simulink model "motorcontrol"  (R2020b)
settings: Solver=FixedStepDiscrete  StartTime=0.0  StopTime=20  FixedStep=Ts.simulink  MaxStep=5e-5  RelTol=1e-3  EnableMultiTasking=on
values from neighbouring files (symbols this model uses):
  dataType = 'single'    [motorcontrol_params.m]
undefined symbols (not defined in the file or in its folder): ControllerMode, ControlMode, ctrlParams, DiscIntNeverNeededParam, inverter, NumBits1, NumBits2, PI_params, pmsm, Slope1, Slope2, Ts
libraries: simulink x14, pid_lib x3
(part 1 of 3)
settings Model: Creator=26046633  LastModifiedBy=26046633
settings SolverCC: ZeroCrossAlgorithm=Adaptive
settings OptimizationCC: DefaultUnderspecifiedDataType=single
settings DebuggingCC: IgnoredZcDiagnostic=none  MultiTaskDSMMsg=none  IntegerOverflowMsg=none  ParameterOverflowMsg=none  ParameterPrecisionLossMsg=none  ParameterTunabilityLossMsg=none
settings RTWCC: Toolchain=MinGW64 | gmake (64-bit Windows)

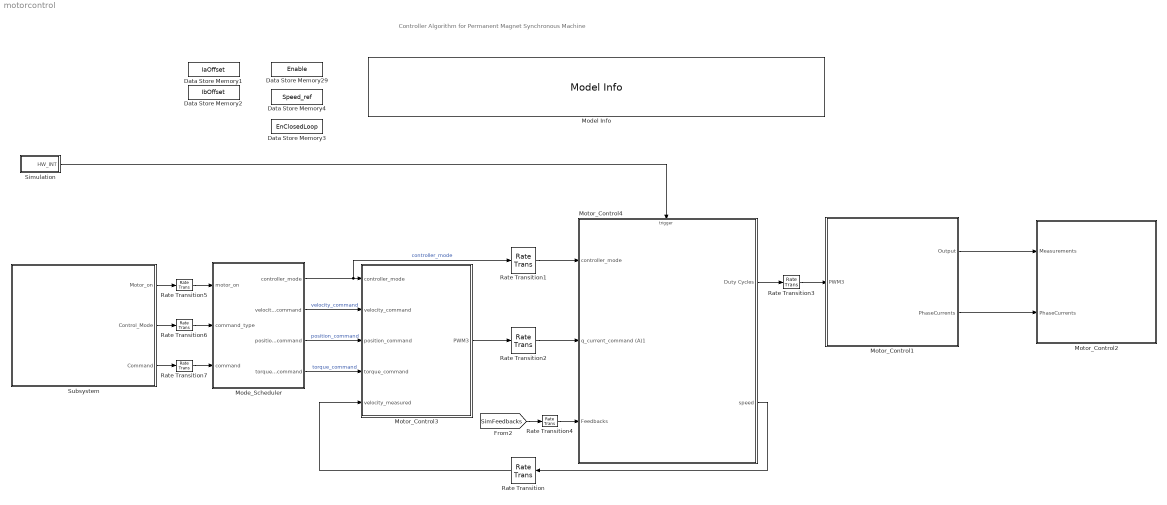
== system motorcontrol ==
  note: Controller Algorithm for Permanent Magnet Synchronous Machine
  Data Store Memory1 : DataStoreMemory  DataStoreName=IaOffset  InitialValue=inverter.CtSensAOffset  ShowAdditionalParam=off
  Data Store Memory2 : DataStoreMemory  DataStoreName=IbOffset  InitialValue=inverter.CtSensBOffset  ShowAdditionalParam=off
  Data Store Memory29 : DataStoreMemory  DataStoreName=Enable  ShowAdditionalParam=off  OutDataTypeStr=boolean
  Data Store Memory3 : DataStoreMemory  DataStoreName=EnClosedLoop  ShowAdditionalParam=off  OutDataTypeStr=boolean
  Data Store Memory4 : DataStoreMemory  DataStoreName=Speed_ref  ShowAdditionalParam=off  OutDataTypeStr=dataType
  Mode_Scheduler : Subsystem  TreatAsAtomicUnit=on  SystemSampleTime=Ts.speed
      mask Display: fprintf('Mode\nScheduler')
  Model Info : simulink/Model-Wide Utilities/Model Info  Frame=on  DisplayStringWithTags=|  HorizontalTextAlignment=Left  LeftAlignmentValue=0.02
      | %<Description>  Model Description: Controller Algorithm for Permanent Magnet Synchronous Motor
      | 
      | %<ModifiedComment> Specifies controller software for Permanent Magnet Synchronous Machine (PMSM) using Field-Oriented Control.
      | 
      | Created By: %<Created>  | Alper Senem [26046633]
      | Last Modification: %<LastModificationDate> | %<LastModifiedBy>
      | Version: %<ModelVersion>
  Motor_Control1 : Subsystem
      settings: RTWSystemCode=Nonreusable function  RTWFcnNameOpts=Use subsystem name
      mask Display: fprintf('Voltage Source Inverter \n\n & PMSM')
  Motor_Control2 : Subsystem
      settings: RTWSystemCode=Nonreusable function  RTWFcnNameOpts=Use subsystem name
      mask Display: fprintf('Measurements')
  Motor_Control3 : Subsystem  TreatAsAtomicUnit=on  SystemSampleTime=Ts.speed
      settings: RTWSystemCode=Nonreusable function  RTWFcnNameOpts=Use subsystem name
      mask Display: fprintf('Motor\nControl')
  Motor_Control4 : Subsystem
      settings: RTWSystemCode=Nonreusable function  RTWFcnNameOpts=Use subsystem name
      mask Display: fprintf('Field Oriented\nControl')
  Rate Transition : RateTransition  Deterministic=off  OutPortSampleTime=Ts.speed
  Rate Transition1 : RateTransition  Deterministic=off  InitialCondition=ControllerMode.SpeedControl  OutPortSampleTime=Ts.pwm
  Rate Transition2 : RateTransition  Deterministic=off  OutPortSampleTime=Ts.pwm
  Rate Transition3 : RateTransition  Deterministic=off  OutPortSampleTime=Ts.inverter
  Rate Transition4 : RateTransition  Deterministic=off  OutPortSampleTime=Ts.pwm
  Rate Transition5 : RateTransition  Integrity=off  Deterministic=off  OutPortSampleTime=Ts.speed
  Rate Transition6 : RateTransition  Integrity=off  Deterministic=off  OutPortSampleTime=Ts.speed
  Rate Transition7 : RateTransition  Deterministic=off  OutPortSampleTime=Ts.speed
  Simulation : Subsystem
  Subsystem : Subsystem  TreatAsAtomicUnit=on  SystemSampleTime=0.01
  wires:
  Motor_Control3/1(PWM3) -> Rate Transition2/1
  Motor_Control1/1(Output) -> Motor_Control2/1(Measurements)
  Motor_Control4/2(speed) -> Rate Transition/1
  Subsystem/3(Command) -> Rate Transition7/1
  Rate Transition/1 -> Motor_Control3/5(velocity_measured)
  Subsystem/2(Control_Mode) -> Rate Transition6/1
  Subsystem/1(Motor_on) -> Rate Transition5/1
  Mode_Scheduler/1(controller_mode) -> Rate Transition1/1, Motor_Control3/1(controller_mode)  "controller_mode"
  Mode_Scheduler/2(velocity_command) -> Motor_Control3/2(velocity_command)  "velocity_command"
  Mode_Scheduler/4(torque_command) -> Motor_Control3/4(torque_command)  "torque_command"
  Mode_Scheduler/3(position_command) -> Motor_Control3/3(position_command)  "position_command"
  Simulation/1(HW_INT) -> Motor_Control4/Trigger
  Motor_Control4/1(Duty Cycles) -> Rate Transition3/1
  Motor_Control1/2(PhaseCurrents) -> Motor_Control2/2(PhaseCurrents)
  Rate Transition3/1 -> Motor_Control1/1(PWM3)
  Rate Transition4/1 -> Motor_Control4/3(Feedbacks)
  Rate Transition2/1 -> Motor_Control4/2(q_current_command (A)1)
  [SimFeedbacks] -> Rate Transition4/1
  Rate Transition1/1 -> Motor_Control4/1(controller_mode)
  Rate Transition5/1 -> Mode_Scheduler/1(motor_on)
  Rate Transition6/1 -> Mode_Scheduler/2(command_type)
  Rate Transition7/1 -> Mode_Scheduler/3(command)

== system motorcontrol/Mode_Scheduler ==
  note: Mode Scheduler
  note: Configures controller mode and controller inputs based on user commands.
  motor_on : Inport
  command_type : Inport  Port=2
  command : Inport  Port=3
  Controller_Mode_Scheduler : Stateflow chart  SystemSampleTime=Ts
  Signal Conversion : SignalConversion  OverrideOpt=on
  Signal Conversion1 : SignalConversion  OverrideOpt=on
  Signal Conversion2 : SignalConversion  OverrideOpt=on
  controller_mode : Outport
  velocity_command : Outport  Port=2
  position_command : Outport  Port=3
  torque_command : Outport  Port=4
  wires:
  Signal Conversion2/1 -> Controller_Mode_Scheduler/3(command)
  Signal Conversion1/1 -> Controller_Mode_Scheduler/2(command_type)
  Signal Conversion/1 -> Controller_Mode_Scheduler/1(motor_on)
  command/1 -> Signal Conversion2/1
  Controller_Mode_Scheduler/4(torque_command) -> torque_command/1
  command_type/1 -> Signal Conversion1/1
  Controller_Mode_Scheduler/3(position_command) -> position_command/1
  motor_on/1 -> Signal Conversion/1
  Controller_Mode_Scheduler/2(velocity_command) -> velocity_command/1
  Controller_Mode_Scheduler/1(controller_mode) -> controller_mode/1

== system motorcontrol/Motor_Control1 ==
  note: Voltage Source Inverter & PMSM
  note: This layer consists ideal 3 phase 2-leg ideal voltage source inverter which generates phase voltages.
      | Also includes PMSM mathematical model
  PWM3 : Inport
  Constant : Constant  Value=0.01  OutDataTypeStr=dataType  SampleTime=Ts.motor
  Inverter : Subsystem  TreatAsAtomicUnit=on  SystemSampleTime=Ts.inverter
  PMSM : Subsystem  SystemSampleTime=Ts.motor  mask(Surface Mount PMSM){Ts=Ts.motor, P=pmsm.p, Rs=pmsm.Rs + inverter.R_board, Ld=pmsm.Ld, Lq=pmsm.Lq, FluxPM=pmsm.FluxPM, J=pmsm.J, B=pmsm.B, Tf=0, idq0=[0 0], theta_init=0, omega_init=0}
      mask prompts: Ts "Sample Time (Ts)"; P "Number of pole pairs"; Rs "Stator resistance per phase (Rs) [Ohm]"; Ld "Stator d-axis inductance(Ld) [H]"; Lq "Stator q-axis inductance(Lq) [H]"; FluxPM "Permanent flux linkage constant"; J "Physical inertia(J) [Kgm^2]"; B "Viscous damping(B) [Nm/rad/s]"; Tf "Static Friction(Tf) [Nm]"; idq0 "Initial d-axis and q-axis current [A,A]"; theta_init "Initial rotor mechanical position [rad]"; omega_init "Initial rotor mechanical speed [rad/s]"
      mask help: Model the dynamics of a three-phase surface mount permanent magnet synchronous motor (PMSM) with sinusoidal back electromotive force.
      mask DialogControl ParamTab Prompt: Parameters
      mask DialogControl Container6 Prompt: Initial Values
      mask Display: fprintf('Surface Mount\n PMSM');
  Output : Outport
  PhaseCurrents : Outport  Port=2
  wires:
  Constant/1 -> PMSM/1(LdTrq)
  PMSM/1(Info) -> Output/1  "info"
  Inverter/1(Vabc) -> PMSM/2(PhaseVolt)  "Vabc"
  PWM3/1 -> Inverter/1(Duty_abc)
  PMSM/2(PhaseCurr) -> PhaseCurrents/1

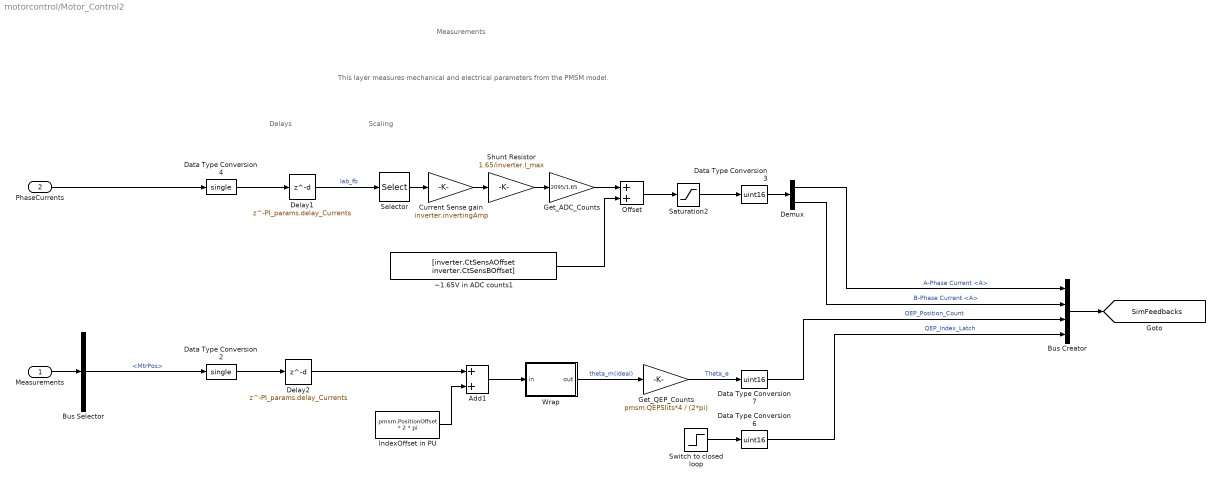
== system motorcontrol/Motor_Control2 ==
  note: Measurements
  note: This layer measures mechanical and electrical parameters from the PMSM model.
  note: Delays
  note: Scaling
  Measurements : Inport
  PhaseCurrents : Inport  Port=2
  Add1 : Sum  RndMeth=Simplest
  Bus Creator : BusCreator  Inputs=4
  Bus Selector : BusSelector  OutputSignals=MtrPos
  Current Sense gain : Gain  Gain=inverter.invertingAmp
  Data Type Conversion2 : DataTypeConversion  OutDataTypeStr=single  RndMeth=Simplest
  Data Type Conversion3 : DataTypeConversion  OutDataTypeStr=uint16
  Data Type Conversion4 : DataTypeConversion  OutDataTypeStr=single  RndMeth=Simplest
  Data Type Conversion6 : DataTypeConversion  OutDataTypeStr=uint16  RndMeth=Simplest
  Data Type Conversion7 : DataTypeConversion  OutDataTypeStr=uint16  RndMeth=Simplest
  Delay1 : Delay  DelayLength=PI_params.delay_Currents
  Delay2 : Delay  DelayLength=PI_params.delay_Currents
  Demux : Demux  Outputs=2
  Get_ADC_Counts : Gain  Gain=2095/1.65  RndMeth=Simplest  OutDataTypeStr=Inherit: Same as input
  Get_QEP_Counts : Gain  Gain=pmsm.QEPSlits*4 / (2*pi)  OutDataTypeStr=uint16  RndMeth=Simplest
  IndexOffset in PU : Constant  Value=pmsm.PositionOffset * 2 * pi  OutDataTypeStr=single  SampleTime=-1
  Offset : Sum  OutDataTypeStr=uint16
  Saturation2 : Saturate  UpperLimit=4095  LowerLimit=0
  Selector : Selector  InputPortWidth=3  IndexOptions=Index vector (dialog)  Indices=[1 2]  OutputSizes=1
  Shunt Resistor : Gain  Gain=1.65/inverter.I_max  RndMeth=Simplest
  Switch to closed loop : Step  Time=0.1  OutDataTypeStr=single  SampleTime=Ts.motor
  Wrap : Subsystem
  ~1.65V in ADC counts1 : Constant  Value=[inverter.CtSensAOffset inverter.CtSensBOffset]  OutDataTypeStr=uint16  SampleTime=-1
  tag scope: SimFeedbacks=global
  wires:
  Wrap/1(out) -> Get_QEP_Counts/1  "theta_m(ideal)"
  Add1/1 -> Wrap/1(in)
  Data Type Conversion6/1 -> Bus Creator/4  "QEP_Index_Latch"
  Data Type Conversion3/1 -> Demux/1
  Switch to closed loop/1 -> Data Type Conversion6/1
  Offset/1 -> Saturation2/1
  Demux/2 -> Bus Creator/2  "B-Phase Current <A>"
  Measurements/1 -> Bus Selector/1
  Data Type Conversion2/1 -> Delay2/1
  Selector/1 -> Current Sense gain/1
  Saturation2/1 -> Data Type Conversion3/1
  Demux/1 -> Bus Creator/1  "A-Phase Current <A>"
  Delay2/1 -> Add1/1
  Current Sense gain/1 -> Shunt Resistor/1
  IndexOffset in PU/1 -> Add1/2
  Get_ADC_Counts/1 -> Offset/1
  Bus Selector/1 -> Data Type Conversion2/1  "<MtrPos>"
  PhaseCurrents/1 -> Data Type Conversion4/1
  Get_QEP_Counts/1 -> Data Type Conversion7/1  "Theta_e"
  Delay1/1 -> Selector/1  "Iab_fb"
  Data Type Conversion7/1 -> Bus Creator/3  "QEP_Position_Count"
  Data Type Conversion4/1 -> Delay1/1
  ~1.65V in ADC counts1/1 -> Offset/2
  Shunt Resistor/1 -> Get_ADC_Counts/1
  Bus Creator/1 -> [SimFeedbacks]

== system motorcontrol/Motor_Control3 ==
  note: This layer executes the control law, and calculates compare values used by the PWM driver.
      | The controller outputs compare values used by the Pulse Width Modulators (PWMs) to generate the phase voltages.
  note: Motor Control
  controller_mode : Inport
  velocity_command : Inport  Port=2
  position_command : Inport  Port=3
  torque_command : Inport  Port=4
  velocity_measured : Inport  Port=5
  Control Modes : Subsystem
  Ground : Ground
  Rate Transition : RateTransition  Deterministic=off  OutPortSampleTime=Ts.speed
  Subsystem1 : Subsystem  mask{FilterConstant=0.01*(Ts.speed/Ts.pwm)}
      mask prompts: FilterConstant "Filter coefficient"
      mask help:
      | Implement an IIR Filter on target hardware by implementing the formula:
      |
      |  y_k = a.x_k + (1-a).y_(k-1)
      |
      | Where, a is the filter coefficient.
      | Lower filter coefficient gives better filtering, but increases the delay in response time.
      mask TypeOptions FilterConstant: Filter_Constant/Value
      mask DialogControl DescGroupVar Prompt: IIR Filter
      mask DialogControl DescTextVar Prompt: Implement an IIR Filter on target hardware by implementing the formula:   y_k = a.x_k + (1-a).y_(k-1)  Where, a is the filter coefficient. Lower filter coefficient gives better filtering, but increases the delay in response time.
      mask Display: fprintf('IIR\n Filter')
  Subsystem2 : Subsystem
  PWM3 : Outport
  wires:
  controller_mode/1 -> Control Modes/1(controller_mode)
  Control Modes/1(PWM3) -> PWM3/1
  Rate Transition/1 -> Control Modes/6(position_measured)
  position_command/1 -> Control Modes/5(position_command)
  torque_command/1 -> Control Modes/4(torque_command)
  Subsystem1/1(y) -> Control Modes/2(velocity_command)  "Speed_ref"
  velocity_command/1 -> Subsystem2/1(Speed_Ref_In)
  Subsystem2/1(Speed_Ref_PU) -> Subsystem1/1(x)  "Speed_Ref"
  velocity_measured/1 -> Subsystem2/2(Speed_Ref_Open), Control Modes/3(velocity_measured)  "Speed_fb"
  Ground/1 -> Rate Transition/1

== system motorcontrol/Motor_Control4 ==
  note: Field Oriented Controller
  note: This layer executes the control law, and calculates compare values used by the PWM driver.
      | The controller outputs compare values used by the Pulse Width Modulators (PWMs) to generate the phase voltages.
  controller_mode : Inport
  q_current_command (A)1 : Inport  Port=2
  Feedbacks : Inport  Port=3
  Trigger : TriggerPort  TriggerType=function-call  VariantControl=Variant  PortDimensions=1
  Bus Selector : BusSelector  OutputSignals=A-Phase Current <A>,B-Phase Current <A>,QEP_Position_Count,QEP_Index_Latch
  Input Scaling : Subsystem
  Inverter (Simulation) : Subsystem
  Mux : Mux  Inputs=2
  Output Scaling1 : Subsystem
  Subsystem : Subsystem
  Duty Cycles : Outport  InitialOutput=0  VectorParamsAs1DForOutWhenUnconnected=off
  speed : Outport  Port=2
  wires:
  Output Scaling1/1(PWM_Duty_Cycles) -> Mux/1
  Mux/1 -> Inverter (Simulation)/1(Inverter Signals)
  Output Scaling1/2(PWM_Enable) -> Mux/2
  Inverter (Simulation)/1(Sim) -> Duty Cycles/1
  controller_mode/1 -> Subsystem/1(controller_mode)
  q_current_command (A)1/1 -> Subsystem/2(q_current_command (A)1)
  Subsystem/1(Out2) -> Output Scaling1/1(Vabc_ref)
  Input Scaling/2(Iab_meas) -> Subsystem/4(Iab_fb)  "Iab_fb"
  Input Scaling/1(Pos) -> Subsystem/3(Pos)  "Position"
  Input Scaling/3(EnClosedLoop) -> Subsystem/5(EnClosedLoop)
  Feedbacks/1 -> Bus Selector/1  "Iab_fb"
  Bus Selector/1 -> Input Scaling/1(Ia_ADC)  "<A-Phase Current <A>>"
  Bus Selector/2 -> Input Scaling/2(Ib_ADC)  "<B-Phase Current <A>>"
  Bus Selector/3 -> Input Scaling/3(QEP_Position_Count)  "<QEP_Position_Count>"
  Bus Selector/4 -> Input Scaling/4(QEP_Index_Latch)  "<QEP_Index_Latch>"
  Input Scaling/4(speed) -> Subsystem/6(speed), speed/1  "Speed"

== system motorcontrol/Simulation ==
  ADCINT1 : simulink/Ports & Subsystems/Function-Call Generator  sample_time=Ts.pwm  numberOfIterations=1  DisallowWideOutput=off
  HW_INT : Outport
  wires:
  ADCINT1/1 -> HW_INT/1

== system motorcontrol/Subsystem ==
  Command_Type : simulink/Sources/Enumerated Constant  OutDataTypeStr=Enum: ControlMode  Value=ControlMode.Speed  SampleTime=-1
  Data Store Write : DataStoreWrite  DataStoreName=Enable
  Data Store Write1 : DataStoreWrite  DataStoreName=Speed_ref
  Data_Type_Float : Subsystem  VariantControl=isequal(dataType, 'single')
  Simulation : Subsystem
  unParse : Subsystem
  Motor_on : Outport
  Control_Mode : Outport  Port=2
  Command : Outport  Port=3
  wires:
  Data_Type_Float/1(Desired Speed) -> Data Store Write1/1, Command/1  "Command"
  unParse/1(Enable_PWM) -> Motor_on/1, Data Store Write/1
  Data_Type_Float/2(Out2) -> unParse/1(Data)
  Simulation/1(Data) -> Data_Type_Float/1(Data)
  Command_Type/1 -> Control_Mode/1  "Control_Mode"

== system motorcontrol/Motor_Control1/Inverter ==
  Duty_abc : Inport
  Average_Value_Inverter : Subsystem
  Constant2 : Constant  Value=inverter.V_dc  OutDataTypeStr=dataType  SampleTime=-1
  Data Type Conversion1 : DataTypeConversion  OutDataTypeStr=dataType  RndMeth=Simplest
  Demux : Demux  Outputs=3
  Inverter_delay : DiscreteTransferFcn  Numerator=[1-exp(-Ts.inverter/(Ts.pwm/2))]  Denominator=[1 -exp(-Ts.inverter/(Ts.pwm/2))]  RndMeth=Simplest
  Mux : Mux  Inputs=3
  Vabc : Outport  VectorParamsAs1DForOutWhenUnconnected=off
  wires:
  Duty_abc/1 -> Data Type Conversion1/1
  Inverter_delay/1 -> Vabc/1
  Data Type Conversion1/1 -> Demux/1
  Demux/2 -> Average_Value_Inverter/2(Vbo)
  Demux/3 -> Average_Value_Inverter/3(Vco)
  Demux/1 -> Average_Value_Inverter/1(Vao)
  Average_Value_Inverter/1(Va) -> Mux/1
  Average_Value_Inverter/3(Vc) -> Mux/3
  Constant2/1 -> Average_Value_Inverter/4(Vdc)
  Mux/1 -> Inverter_delay/1  "Vabc"
  Average_Value_Inverter/2(Vb) -> Mux/2

== system motorcontrol/Motor_Control1/PMSM ==
  LdTrq : Inport
  PhaseVolt : Inport  Port=2
  Subsystem : Subsystem
  Info : Outport  VectorParamsAs1DForOutWhenUnconnected=off
  PhaseCurr : Outport  Port=2  VectorParamsAs1DForOutWhenUnconnected=off
  wires:
  LdTrq/1 -> Subsystem/1(LdTrq)
  PhaseVolt/1 -> Subsystem/2(PhaseVolt)
  Subsystem/2(PhaseCurr) -> PhaseCurr/1
  Subsystem/1(Info) -> Info/1

== system motorcontrol/Motor_Control2/Wrap ==
  in : Inport
  Constant2 : Constant  Value=2*pi  OutDataTypeStr=single  SampleTime=-1
  Mod : Math  Operator=mod  SaturateOnIntegerOverflow=on
  out : Outport  VectorParamsAs1DForOutWhenUnconnected=off
  wires:
  Mod/1 -> out/1
  Constant2/1 -> Mod/2
  in/1 -> Mod/1

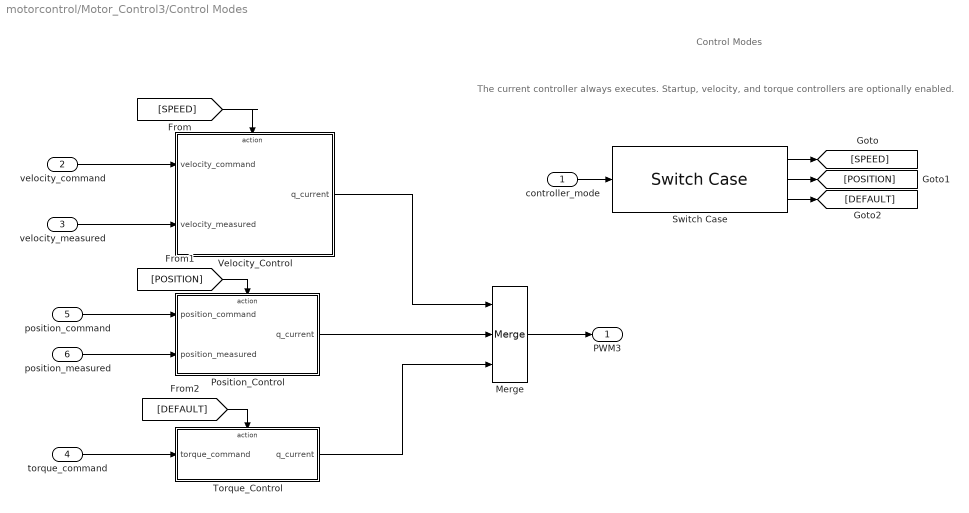
== system motorcontrol/Motor_Control3/Control Modes ==
  note: The current controller always executes. Startup, velocity, and torque controllers are optionally enabled.
  note: Control Modes
  controller_mode : Inport
  velocity_command : Inport  Port=2
  velocity_measured : Inport  Port=3
  torque_command : Inport  Port=4
  position_command : Inport  Port=5
  position_measured : Inport  Port=6
  Merge : Merge  Inputs=3
  Position_Control : Subsystem  TreatAsAtomicUnit=on
  Switch Case : SwitchCase  CaseConditions={ControllerMode.SpeedControl,ControllerMode.PositionControl}
  Torque_Control : Subsystem  TreatAsAtomicUnit=on
  Velocity_Control : Subsystem
  PWM3 : Outport
  wires:
  velocity_measured/1 -> Velocity_Control/2(velocity_measured)
  Position_Control/1(q_current) -> Merge/2
  Velocity_Control/1(q_current) -> Merge/1
  Torque_Control/1(q_current) -> Merge/3
  torque_command/1 -> Torque_Control/1(torque_command)
  position_command/1 -> Position_Control/1(position_command)
  Switch Case/1 -> [SPEED]
  Switch Case/2 -> [POSITION]
  Switch Case/3 -> [DEFAULT]
  [SPEED] -> Velocity_Control/Action
  [POSITION] -> Position_Control/Action
  [DEFAULT] -> Torque_Control/Action
  position_measured/1 -> Position_Control/2(position_measured)
  velocity_command/1 -> Velocity_Control/1(velocity_command)
  controller_mode/1 -> Switch Case/1
  Merge/1 -> PWM3/1

== system motorcontrol/Motor_Control3/Subsystem1 ==
  x : Inport
  Add : Sum
  Add1 : Sum  Inputs=-+
  Constant : Constant  OutDataTypeStr=dataType  SampleTime=-1
  Data Type Duplicate : DataTypeDuplicate  NumInputPorts=3
  Filter_Constant : Constant  Value=FilterConstant  OutDataTypeStr=dataType  SampleTime=-1
  Product : Product
  Product1 : Product
  Unit Delay : UnitDelay  SampleTime=-1  HasFrameUpgradeWarning=on
  y : Outport
  wires:
  x/1 -> Product/1, Data Type Duplicate/1
  Filter_Constant/1 -> Product/2, Add1/1, Data Type Duplicate/2
  Product/1 -> Add/1
  Add/1 -> y/1, Unit Delay/1
  Product1/1 -> Add/2
  Unit Delay/1 -> Product1/2
  Add1/1 -> Product1/1
  Constant/1 -> Data Type Duplicate/3, Add1/2

== system motorcontrol/Motor_Control3/Subsystem2 ==
  Speed_Ref_In : Inport
  Speed_Ref_Open : Inport  Port=2
  AND : Logic  IconShape=distinctive  AllPortsSameDT=off  OutDataTypeStr=boolean
  Data Store Read : DataStoreRead  DataStoreName=EnClosedLoop
  Data Store Read1 : DataStoreRead  DataStoreName=Enable
  RPM to rad/s : Gain  Gain=2 * pi / 60  RndMeth=Simplest  OutDataTypeStr=Inherit: Same as input
  Switch : Switch  Criteria=u2 > Threshold  Threshold=0.5  OutDataTypeStr=single
  Speed_Ref_PU : Outport
  wires:
  RPM to rad/s/1 -> Switch/1
  Data Store Read1/1 -> AND/2
  Switch/1 -> Speed_Ref_PU/1
  Speed_Ref_Open/1 -> Switch/3
  Speed_Ref_In/1 -> RPM to rad/s/1
  Data Store Read/1 -> AND/1
  AND/1 -> Switch/2

== system motorcontrol/Motor_Control4/Input Scaling ==
  note: QEP
  note: Position & Speed Measurements
  note: Current Measurements
  Ia_ADC : Inport
  Ib_ADC : Inport  Port=2
  QEP_Position_Count : Inport  Port=3
  QEP_Index_Latch : Inport  Port=4
  " Calculate Position and Speed" : Subsystem
  Calculate Phase Currents : Subsystem
  IndexOffset : Constant  Value=pmsm.PositionOffset * 2 * pi  OutDataTypeStr=dataType  SampleTime=-1
  Pos : Outport
  Iab_meas : Outport  Port=2
  EnClosedLoop : Outport  Port=3
  speed : Outport  Port=4  OutDataTypeStr=single
  wires:
  " Calculate Position and Speed"/3(IndexFound) -> EnClosedLoop/1
  IndexOffset/1 -> " Calculate Position and Speed"/3(Offset)
  QEP_Index_Latch/1 -> " Calculate Position and Speed"/2(QEP_Index_Latch)
  Ib_ADC/1 -> Calculate Phase Currents/2(Ib_ADC)
  Ia_ADC/1 -> Calculate Phase Currents/1(Ia_ADC)
  " Calculate Position and Speed"/1(Theta_e) -> Pos/1
  QEP_Position_Count/1 -> " Calculate Position and Speed"/1(QEP_Position_Count)
  Calculate Phase Currents/1(Iab_meas) -> Iab_meas/1  "Iab_fb"
  " Calculate Position and Speed"/2(speed) -> speed/1

== system motorcontrol/Motor_Control4/Inverter (Simulation) ==
  Inverter Signals : Inport
  Data Type Duplicate : DataTypeDuplicate
  Demux : Demux
  Mux : Mux  Inputs=3
  Mux2 : Mux  Inputs=3
  Switch1 : Switch  Threshold=0.5  RndMeth=Simplest
  stop : Constant  Value=0  OutDataTypeStr=Inherit: Inherit via back propagation
  Sim : Outport  VectorParamsAs1DForOutWhenUnconnected=off
  wires:
  Demux/3 -> Mux/3
  Demux/2 -> Mux/2
  Demux/1 -> Mux/1
  Mux/1 -> Switch1/1, Data Type Duplicate/1  "PWM Duty Cycles"
  Demux/4 -> Switch1/2  "PWM Enable"
  Inverter Signals/1 -> Demux/1
  Switch1/1 -> Sim/1
  Mux2/1 -> Switch1/3
  stop/1 -> Mux2/2, Mux2/3, Mux2/1, Data Type Duplicate/2

== system motorcontrol/Motor_Control4/Output Scaling1 ==
  Vabc_ref : Inport  OutDataTypeStr=dataType
  Constant : Constant  Value=0.5  OutDataTypeStr=dataType  SampleTime=-1
  Data Type Conversion : DataTypeConversion  OutDataTypeStr=dataType
  Enable : DataStoreRead  DataStoreName=Enable
  One_by_Two : Gain  Gain=1/ (2 * inverter.V_dc)  OutDataTypeStr=dataType  RndMeth=Simplest
  Sum : Sum  Inputs=|++  OutDataTypeStr=dataType
  PWM_Duty_Cycles : Outport  OutDataTypeStr=dataType
  PWM_Enable : Outport  Port=2
  wires:
  One_by_Two/1 -> Sum/1
  Sum/1 -> PWM_Duty_Cycles/1  "PWM_Duty_Cycles"
  Vabc_ref/1 -> One_by_Two/1
  Constant/1 -> Sum/2
  Enable/1 -> Data Type Conversion/1  "PWM_En"
  Data Type Conversion/1 -> PWM_Enable/1

== system motorcontrol/Motor_Control4/Subsystem ==
  controller_mode : Inport
  q_current_command (A)1 : Inport  Port=2
  Pos : Inport  Port=3
  Iab_fb : Inport  Port=4
  EnClosedLoop : Inport  Port=5
  speed : Inport  Port=6
  Closed_Loop : Subsystem
  NOT : Logic  Operator=NOT  IconShape=distinctive  AllPortsSameDT=off  OutDataTypeStr=boolean
  Open Loop Start-Up : Subsystem
  Switch4 : Switch  Threshold=0.5  OutDataTypeStr=Inherit: Inherit via back propagation  RndMeth=Simplest
  Out2 : Outport
  wires:
  Open Loop Start-Up/1(Vabc) -> Switch4/3
  EnClosedLoop/1 -> Switch4/2, NOT/1, Closed_Loop/Enable
  controller_mode/1 -> Closed_Loop/1(controller_mode)
  q_current_command (A)1/1 -> Closed_Loop/2(q_current_command (A)1)
  Closed_Loop/1(Out1) -> Switch4/1
  NOT/1 -> Open Loop Start-Up/Enable
  Switch4/1 -> Out2/1
  Pos/1 -> Closed_Loop/3(Feedback)
  Iab_fb/1 -> Closed_Loop/4(Iab_fb)
  speed/1 -> Closed_Loop/5(Speed)

== system motorcontrol/Subsystem/Data_Type_Float ==
  Data : Inport
  Data Type Conversion2 : DataTypeConversion  OutDataTypeStr=uint16  RndMeth=Simplest
  Demux : Demux  Outputs=2
  Desired Speed : Outport
  Out2 : Outport  Port=2
  wires:
  Demux/2 -> Data Type Conversion2/1
  Data Type Conversion2/1 -> Out2/1
  Demux/1 -> Desired Speed/1
  Data/1 -> Demux/1

== system motorcontrol/Subsystem/Simulation ==
  Data Type Conversion2 : DataTypeConversion  OutDataTypeStr=dataType  RndMeth=Simplest
  Data_Type_Float : Subsystem  VariantControl=isequal(dataType, 'single')
  Enable : Constant  OutDataTypeStr=uint16  SampleTime=-1
  Parse : Subsystem
  Reversal : Step  Time=6  OutDataTypeStr=dataType
  Speed_Ref_Final (rpm) : Constant  Value=-1000  OutDataTypeStr=dataType  SampleTime=-1
  Speed_Ref_Init (rpm) : Step  Time=4  Before=300  After=1000  OutDataTypeStr=dataType
  Switch : Switch  Criteria=u2 > Threshold
  Data : Outport
  wires:
  Data Type Conversion2/1 -> Data_Type_Float/1(In1)
  Switch/1 -> Data Type Conversion2/1
  Parse/1(Data) -> Data_Type_Float/2(In2)
  Enable/1 -> Parse/1(Enable_PWM)
  Reversal/1 -> Switch/2
  Speed_Ref_Init (rpm)/1 -> Switch/3
  Speed_Ref_Final (rpm)/1 -> Switch/1
  Data_Type_Float/1(Data) -> Data/1

== system motorcontrol/Subsystem/unParse ==
  Data : Inport
  Bitwise Operator : simulink/Logic and Bit Operations/Bitwise Operator  logicop=AND  UseBitMask=on  BitMask=hex2dec('0001')  BitMaskRealWorld=Stored Integer
  Data Type Conversion3 : DataTypeConversion  OutDataTypeStr=boolean  RndMeth=Simplest
  Enable_PWM : Outport
  wires:
  Data Type Conversion3/1 -> Enable_PWM/1
  Bitwise Operator/1 -> Data Type Conversion3/1
  Data/1 -> Bitwise Operator/1

== system motorcontrol/Motor_Control1/Inverter/Average_Value_Inverter ==
  Vao : Inport
  Vbo : Inport  Port=2
  Vco : Inport  Port=3
  Vdc : Inport  Port=4
  Gain : Gain  Gain=1/3  RndMeth=Simplest  OutDataTypeStr=Inherit: Same as input
  Product : Product  RndMeth=Simplest  OutDataTypeStr=Inherit: Same as first input
  Product1 : Product  RndMeth=Simplest  OutDataTypeStr=Inherit: Same as first input
  Product2 : Product  RndMeth=Simplest  OutDataTypeStr=Inherit: Same as first input
  Sum1 : Sum  Inputs=|++--  RndMeth=Simplest  OutDataTypeStr=Inherit: Same as first input
  Sum2 : Sum  Inputs=|++--  RndMeth=Simplest  OutDataTypeStr=Inherit: Same as first input
  Sum3 : Sum  Inputs=|++--  RndMeth=Simplest  OutDataTypeStr=Inherit: Same as first input
  Va : Outport  VectorParamsAs1DForOutWhenUnconnected=off
  Vb : Outport  Port=2  VectorParamsAs1DForOutWhenUnconnected=off
  Vc : Outport  Port=3  VectorParamsAs1DForOutWhenUnconnected=off
  wires:
  Vbo/1 -> Sum2/4, Sum3/3, Sum1/2, Sum1/1
  Vco/1 -> Sum2/1, Sum2/2, Sum1/3, Sum3/4
  Product/1 -> Va/1  "Va"
  Sum3/1 -> Product/1
  Vdc/1 -> Gain/1
  Sum1/1 -> Product1/1
  Product2/1 -> Vc/1  "Vb"
  Vao/1 -> Sum2/3, Sum1/4, Sum3/2, Sum3/1
  Sum2/1 -> Product2/1
  Gain/1 -> Product2/2, Product1/2, Product/2
  Product1/1 -> Vb/1  "Vb"

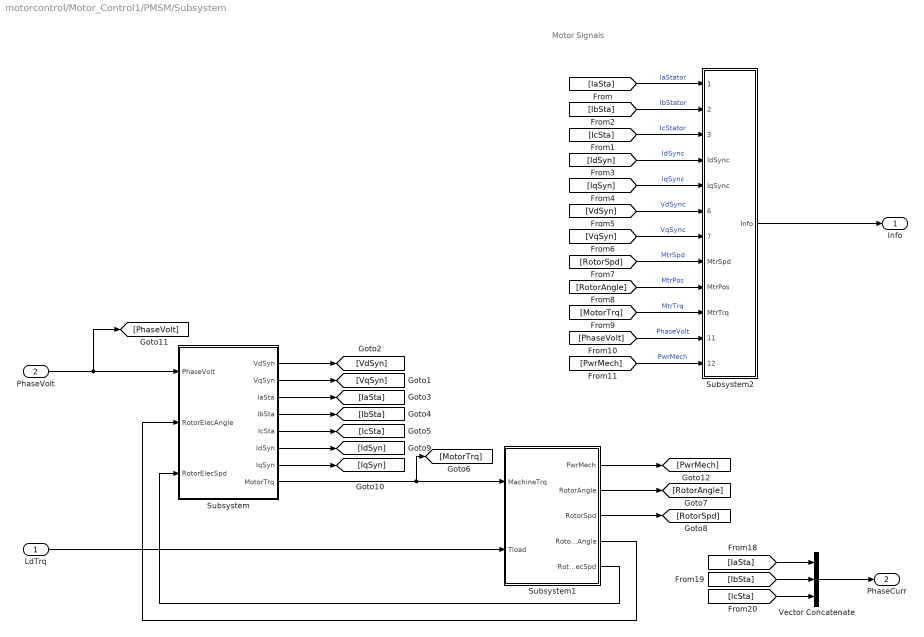
== system motorcontrol/Motor_Control1/PMSM/Subsystem ==
  note: Motor Signals
  LdTrq : Inport
  PhaseVolt : Inport  Port=2
  Subsystem : Subsystem
  Subsystem1 : Subsystem
  Subsystem2 : Subsystem
  Vector Concatenate : Concatenate  NumInputs=3
  Info : Outport  VectorParamsAs1DForOutWhenUnconnected=off
  PhaseCurr : Outport  Port=2  Unit=A  VectorParamsAs1DForOutWhenUnconnected=off
  wires:
  Subsystem/1(VdSyn) -> [VdSyn]
  LdTrq/1 -> Subsystem1/2(Tload)
  Subsystem/4(IbSta) -> [IbSta]
  Subsystem/8(MotorTrq) -> Subsystem1/1(MachineTrq), [MotorTrq]
  [IdSyn] -> Subsystem2/4(IdSync)  "IdSync"
  [IaSta] -> Vector Concatenate/1
  [IaSta] -> Subsystem2/1(IaStator)  "IaStator"
  [IcSta] -> Subsystem2/3(IcStator)  "IcStator"
  [VqSyn] -> Subsystem2/7(VqSync)  "VqSync"
  [IbSta] -> Subsystem2/2(IbStator)  "IbStator"
  [IqSyn] -> Subsystem2/5(IqSync)  "IqSync"
  [PhaseVolt] -> Subsystem2/11(PhaseVolt)  "PhaseVolt"
  [RotorAngle] -> Subsystem2/9(MtrPos)  "MtrPos"
  [PwrMech] -> Subsystem2/12(PwrMech)  "PwrMech"
  [IbSta] -> Vector Concatenate/2
  Subsystem/3(IaSta) -> [IaSta]
  Subsystem1/4(RotorElecAngle) -> Subsystem/2(RotorElecAngle)
  [MotorTrq] -> Subsystem2/10(MtrTrq)  "MtrTrq"
  Subsystem/5(IcSta) -> [IcSta]
  Subsystem1/5(RotorElecSpd) -> Subsystem/3(RotorElecSpd)
  Vector Concatenate/1 -> PhaseCurr/1
  Subsystem1/2(RotorAngle) -> [RotorAngle]
  Subsystem/6(IdSyn) -> [IdSyn]
  Subsystem2/1(Info) -> Info/1
  Subsystem1/3(RotorSpd) -> [RotorSpd]
  [IcSta] -> Vector Concatenate/3
  Subsystem/2(VqSyn) -> [VqSyn]
  Subsystem1/1(PwrMech) -> [PwrMech]
  PhaseVolt/1 -> [PhaseVolt], Subsystem/1(PhaseVolt)
  Subsystem/7(IqSyn) -> [IqSyn]
  [RotorSpd] -> Subsystem2/8(MtrSpd)  "MtrSpd"
  [VdSyn] -> Subsystem2/6(VdSync)  "VdSync"

== system motorcontrol/Motor_Control3/Control Modes/Position_Control ==
  note: The controller regulates motor position using rotor position feedback compared to a commanded position.
      | The output of the controller is the quadrature-winding current command which is directly proportional to the electromagnetic torque of the motor.
      | Since the motor being controlled is a Permanent Magnet Synchronous Machine, the rotor flux linkage is fixed (determined by the magnets),
      | hence the commanded direct-winding current is always zero.
  note: Position Controller
  position_command : Inport
  position_measured : Inport  Port=2
  Action Port : ActionPort  InitializeStates=reset  ActionPortLabel=case [ PositionControl ]:
      settings: AttributesFormatString=----------------------------\nStates: %<InitializeStates>
  Isolate_For_Merge : SignalConversion  OverrideOpt=off
  Sum2 : Sum  Inputs=|+-
  q_current : Outport
  wires:
  position_measured/1 -> Sum2/2  "position_measured"
  position_command/1 -> Sum2/1  "position_command"
  Sum2/1 -> Isolate_For_Merge/1  "position_error"
  Isolate_For_Merge/1 -> q_current/1

== system motorcontrol/Motor_Control3/Control Modes/Torque_Control ==
  note: The output of the controller is the quadrature-winding current command which is directly proportional to the electromagnetic torque of the motor.
      | In this configuration, the torque command is just the current command. An additional gain term could be added to translate current to torque
      | based on know motor parameters.
  note: Torque Controller
  torque_command : Inport
  Action Port : ActionPort  ActionPortLabel=default:
      settings: AttributesFormatString=----------------------------\nStates: %<InitializeStates>
  q_current : Outport
  wires:
  torque_command/1 -> q_current/1

== system motorcontrol/Motor_Control3/Control Modes/Velocity_Control ==
  note: The controller regulates motor velocity using rotor velocity feedback compared to a commanded velocity.
      | The output of the controller is the quadrature-winding current command which is directly proportional to the electromagnetic torque of the motor.
      | Since the motor being controlled is a Permanent Magnet Synchronous Machine, the rotor flux linkage is fixed (determined by the magnets),
      | hence the commanded direct-winding current is always zero.
  note: Velocity Controller
  velocity_command : Inport
  velocity_measured : Inport  Port=2
  Action Port : ActionPort  InitializeStates=reset  ActionPortLabel=case [ SpeedControl ]:
      settings: AttributesFormatString=----------------------------\nStates: %<InitializeStates>
  Constant : Constant  Value=PI_params.Kp_speed  OutDataTypeStr=dataType  SampleTime=-1
  Constant1 : Constant  Value=PI_params.Ki_speed  OutDataTypeStr=dataType  SampleTime=-1
  Data Store Read1 : DataStoreRead  DataStoreName=Enable
  Isolate_For_Merge : SignalConversion  OverrideOpt=off
  Ki2 : Constant  Value=0  OutDataTypeStr=dataType  SampleTime=-1
  Logical Operator : Logic  Operator=NOT  IconShape=distinctive  AllPortsSameDT=off  OutDataTypeStr=boolean
  Rotor_Speed_Control : pid_lib/PID Controller  Controller=PI  Form=Parallel  TimeDomain=Discrete-time  UseExternalTs=off  SampleTime=-1  IntegratorMethod=Forward Euler  FilterMethod=Forward Euler  ControllerParametersSource=external  P=ctrlParams.Velocity_P  I=ctrlParams.Velocity_I  D=0  UseFilter=on  N=100  TunerSelectOption=Transfer Function Based (PID Tuner App)  InitialConditionSource=external  InitialConditionForIntegrator=0  InitialConditionForFilter=0  DifferentiatorICPrevScaledInput=0  ExternalReset=level  TrackingMode=off  Kt=1  LimitOutput=on  SatLimitsSource=internal  UpperSaturationLimit=inverter.I_max  LowerSaturationLimit=-inverter.I_max  LinearizeAsGain=off  AntiWindupMode=clamping  Kb=0  POutMin=[]  POutMax=[]  IOutMin=[]  IOutMax=[]  DOutMin=[]  DOutMax=[]  NOutMin=[]  NOutMax=[]  SumOutMin=[]  SumOutMax=[]  SaturationOutMin=[]  SaturationOutMax=[]  PParamMin=[]  PParamMax=[]  IParamMin=[]  IParamMax=[]  DParamMin=[]  DParamMax=[]  NParamMin=[]  NParamMax=[]  KbParamMin=[]  KbParamMax=[]  KtParamMin=[]  KtParamMax=[]  KbOutMin=[]  KbOutMax=[]  KtOutMin=[]  KtOutMax=[]  IntegratorOutMin=[]  IntegratorOutMax=[]  FilterOutMin=[]  FilterOutMax=[]  SumI1OutMin=[]  SumI1OutMax=[]  SumI2OutMin=[]  SumI2OutMax=[]  SumI3OutMin=[]  SumI3OutMax=[]  SumI4OutMin=[]  SumI4OutMax=[]  SumDOutMin=[]  SumDOutMax=[]  DifferentiatorOutMin=[]  DifferentiatorOutMax=[]  FilterDiffOutCoefMin=[]  FilterDiffOutCoefMax=[]  ReciprocalOutMin=[]  ReciprocalOutMax=[]  SumDenOutMin=[]  SumDenOutMax=[]  SumNumOutMin=[]  SumNumOutMax=[]  DivideOutMin=[]  DivideOutMax=[]  UdiffTsProdOutMin=[]  UdiffTsProdOutMax=[]  NTsProdOutMin=[]  NTsProdOutMax=[]  UintegralTsProdOutMin=[]  UintegralTsProdOutMax=[]  UngainTsProdOutMin=[]  UngainTsProdOutMax=[]  IntegratorContinuousStateAttributes=''  IntegratorStateMustResolveToSignalObject=off  IntegratorRTWStateStorageClass=Auto  FilterContinuousStateAttributes=''  FilterStateMustResolveToSignalObject=off  FilterRTWStateStorageClass=Auto  ParallelPVariant=ExternalParameters  IdealPVariant=Disabled  IVariant=ExternalParameters  DVariant=Disabled  IntegratorVariant=Discrete  SatVariant=Enabled  AWVariant=DiscClampingParallel  PCopyVariant=Disabled  TRVariant=Disabled  FdbkBlocksVariant=Forward  IdealPFdbkVariant=Disabled  SatFdbkVariant=Disabled  DerivativeFilterVariant=Disabled  NVariant=Disabled  NCopyVariant=Disabled_SignalSpec  FilterICVariant=Disabled  IntegratorICVariant=ExternalICs  ExternalResetVariant=ExternalReset  TRSumVariant=Passthrough  SumFdbkVariant=Disabled  SumVariant=Sum_PI  TsampFilterVariant=InternalTs  TsampNgainVariant=Passthrough  TsampIntegralVariant=Passthrough  ExternalSaturationOutDataTypeStr=Inherit: Same as second input
  Sum2 : Sum  Inputs=|+-
  q_current : Outport
  wires:
  velocity_measured/1 -> Sum2/2  "velocity_measured"
  Sum2/1 -> Rotor_Speed_Control/1  "velocity_error"
  Rotor_Speed_Control/1 -> Isolate_For_Merge/1  "quadrature_current_command"
  velocity_command/1 -> Sum2/1  "velocity_command"
  Isolate_For_Merge/1 -> q_current/1
  Constant/1 -> Rotor_Speed_Control/2
  Constant1/1 -> Rotor_Speed_Control/3
  Data Store Read1/1 -> Logical Operator/1
  Logical Operator/1 -> Rotor_Speed_Control/4
  Ki2/1 -> Rotor_Speed_Control/5

== system motorcontrol/Motor_Control4/Input Scaling/ Calculate Position and Speed ==
  QEP_Position_Count : Inport
  QEP_Index_Latch : Inport  Port=2
  Offset : Inport  Port=3
  Data Store Write : DataStoreWrite  DataStoreName=EnClosedLoop
  Delay : Delay  DelayLength=1
  IndexFinder : Subsystem
  NOT : Logic  Operator=NOT  AllPortsSameDT=off  OutDataTypeStr=boolean
  Subsystem : Subsystem  mask{FilterConstant=0.01}
      mask prompts: FilterConstant "Filter coefficient"
      mask help:
      | Implement an IIR Filter on target hardware by implementing the formula:
      |
      |  y_k = a.x_k + (1-a).y_(k-1)
      |
      | Where, a is the filter coefficient.
      | Lower filter coefficient gives better filtering, but increases the delay in response time.
      mask TypeOptions FilterConstant: Filter_Constant/Value
      mask DialogControl DescGroupVar Prompt: IIR Filter
      mask DialogControl DescTextVar Prompt: Implement an IIR Filter on target hardware by implementing the formula:   y_k = a.x_k + (1-a).y_(k-1)  Where, a is the filter coefficient. Lower filter coefficient gives better filtering, but increases the delay in response time.
      mask Display: fprintf('IIR\n Filter')
  Subsystem1 : Subsystem  mask{DelayLength=20, SampleTimeAsync=Ts.pwm}
      mask prompts: DelayLength "Delays for speed calculation (number of samples):"; SampleTimeAsync "Block Sample Time (s):"
      mask DialogControl DescGroupVar Prompt: Speed Measurement
      mask DialogControl DescTextVar Prompt: Compute the speed from the rotor angular position. Output speed unit is RPM, input position unit is radians.
      mask Display:
      | color('black');
      | port_label('input' , 1 , '\theta' , 'texmode','on');
      | port_label('output',1,'\omega','texmode','on');
      | fprintf('Speed\n Measurement');
  Subsystem2 : Subsystem  mask(Quadrature Decoder){EncoderSlitsPerRevolution=pmsm.QEPSlits, EncoderCountsPerSlit=4, CounterSize=16 bits}
      mask prompts: EncoderSlitsPerRevolution "Encoder Slits:"; EncoderCountsPerSlit "Encoder counts per slit:"; CounterSize "Counter size:"
      mask help:
      | Compute the position of quadrature encoder.
      |
      | Cnt port accepts the quadrature encoder counter value. Idx port is enabled when the External index count is checked. Idx port accepts the counter value at last index pulse. The block only accepts scalar unsigned integer based on the Counter size parameter.
      mask TypeOptions CounterSize: 8 bits | 16 bits | 32 bits
      mask DialogControl DescTextVar Prompt: Compute the position of quadrature encoder.
      mask DialogControl Control2 Prompt: Cnt ports accepts the quadrature encoder counter value. Idx port is enabled when the external index count is checked. Idx port accepts the counter value at last index pulse. The block only accepts scalar unsigned integer based on the Counter size parameter.
      mask Display:
      | color('black');
      | port_label('input',1,'Cnt','interpreter','tex');
      | port_label('output',1,'\theta_m','interpreter','tex');
      | fprintf('Quadrature\nDecoder');
      | port_label('input',2,'Idx');
  Subsystem3 : Subsystem  mask{mechOffsetIn=0, maxAngleIn=2*pi, NrPP=pmsm.p}
      mask prompts: mechOffsetIn "Mechanical offset:"; maxAngleIn "Maximum input angle:"; NrPP "Number of pole pairs:"
      mask DialogControl DescGroupVar Prompt: Mechanical to Electrical Position
      mask DialogControl DescTextVar Prompt: Compute electrical position of the rotor based on mechanical position.
      mask Display:
      | port_label('input',1, '\theta_m','texmode','on');
      | port_label('input',2, 'Offset','texmode','on');
      | port_label('input',1, '\theta_e','texmode','on');
      | fprintf('Mech2Elec\n Position');
  Theta_e : Outport  VectorParamsAs1DForOutWhenUnconnected=off
  speed : Outport  Port=2  VectorParamsAs1DForOutWhenUnconnected=off
  IndexFound : Outport  Port=3  InitialOutput=0  VectorParamsAs1DForOutWhenUnconnected=off
  wires:
  QEP_Index_Latch/1 -> Subsystem2/2(IndexCount), IndexFinder/1(In1)
  IndexFinder/1(Out1) -> Delay/1, IndexFound/1, Data Store Write/1
  NOT/1 -> IndexFinder/Enable
  Delay/1 -> NOT/1
  Subsystem/1(y) -> speed/1
  Offset/1 -> Subsystem3/2(Offset)
  Subsystem2/1(Position) -> Subsystem1/1(Position), Subsystem3/1(ϴm)
  QEP_Position_Count/1 -> Subsystem2/1(Count)
  Subsystem3/1(ϴe) -> Theta_e/1
  Subsystem1/1(Speed) -> Subsystem/1(x)  "speed_meas"

== system motorcontrol/Motor_Control4/Input Scaling/Calculate Phase Currents ==
  Ia_ADC : Inport
  Ib_ADC : Inport  Port=2
  Add : Sum  Inputs=-+
  Current Sense Gain : Gain  Gain=inverter.invertingAmp * inverter.I_max /1.65  RndMeth=Simplest  OutDataTypeStr=Inherit: Same as input
  Data Store Read1 : DataStoreRead  DataStoreName=IaOffset
  Data Store Read2 : DataStoreRead  DataStoreName=IbOffset
  Data Type Conversion : DataTypeConversion  OutDataTypeStr=int32  ConvertRealWorld=Stored Integer (SI)  RndMeth=Simplest
  Get_ADC_Volt : Gain  Gain=1.65/2048  OutDataTypeStr=dataType  RndMeth=Simplest
  Mux : Mux  Inputs=2
  Mux1 : Mux  Inputs=2
  Iab_meas : Outport  VectorParamsAs1DForOutWhenUnconnected=off
  wires:
  Current Sense Gain/1 -> Iab_meas/1
  Get_ADC_Volt/1 -> Current Sense Gain/1
  Mux1/1 -> Add/1
  Data Store Read2/1 -> Mux1/2
  Data Store Read1/1 -> Mux1/1
  Mux/1 -> Data Type Conversion/1
  Ib_ADC/1 -> Mux/2
  Ia_ADC/1 -> Mux/1
  Add/1 -> Get_ADC_Volt/1
  Data Type Conversion/1 -> Add/2

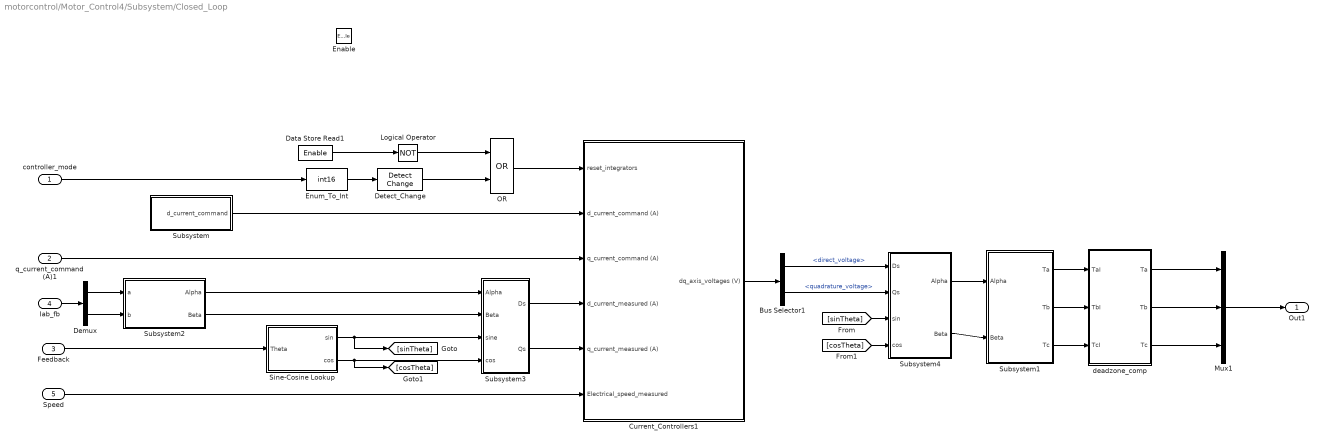
== system motorcontrol/Motor_Control4/Subsystem/Closed_Loop ==
  controller_mode : Inport
  q_current_command (A)1 : Inport  Port=2
  Feedback : Inport  Port=3
  Iab_fb : Inport  Port=4
  Speed : Inport  Port=5
  Enable : EnablePort  StatesWhenEnabling=reset
  Bus Selector1 : BusSelector  OutputSignals=direct_voltage,quadrature_voltage
  Current_Controllers1 : Subsystem  Description=|
      | Linear Current Controllers
      | 
      | PID Blocks used for Control Design of Current Loop controllers.
  Data Store Read1 : DataStoreRead  DataStoreName=Enable
  Demux : Demux  Outputs=2
  Detect_Change : simulink/Logic and Bit Operations/Detect Change  vinit=0  OutDataTypeStr=uint8
  Enum_To_Int : DataTypeConversion  OutDataTypeStr=int16
  Logical Operator : Logic  Operator=NOT  IconShape=distinctive  AllPortsSameDT=off  OutDataTypeStr=boolean
  Mux1 : Mux  Inputs=3
  OR : Logic  Operator=OR  AllPortsSameDT=off  OutDataTypeStr=boolean
  Sine-Cosine Lookup : Subsystem  mask{N_points=1024}
      mask prompts: N_points "Number of data points for lookup table:"
      mask init:
      | this = get_param(gcbh,'Object');
      | 
      | points = eval(this.N_points);
      | 
      | dlgSett.points = 125*floor(points/125);
      | 
      | dlgSett.Offset = uint16(dlgSett.points/5);
      | 
      | dlgSett.N_points = 4*dlgSett.Offset;
      | N_points = dlgSett.N_points;
      | 
      | theta = linspace(0,2*pi,N_points+1);
      | dlgSett.size = 5*dlgSett.Offset+2;
      | dlgSett.sin_table = zeros(1,dlgSett.size);
      | dlgSett.sin_table(1:N_points+1) = sin(theta);
      | dlgSett.sin_table(N_points+2:dlgSett.size) = dlgSett.sin_table(2:0.25*N_points+2);
      | 
      | dlgSett.N_points = double(dlgSett.N_points);
      | dlgSett.index_gain = dlgSett.N_points;
      | dlgSett.UpperSatLimit = 1;
      | dlgSett.UpperSatLimit = 2*pi;
      mask DialogControl DescGroupVar Prompt: Sine-Cosine Lookup
      mask DialogControl DescTextVar Prompt: Implement sine and cosine functions using a lookup table approach for optimized performance on target hardware.
      mask Display: fprintf('Sin-Cos\n LUT');
  Subsystem : Subsystem
  Subsystem1 : Subsystem  mask(Space Vector Generator){}
      mask help:
      | <p>Generate space vector modulation signals from stator reference voltages described by  &alpha;-&beta; components.
      | <br><br>
      | The block accepts V<sub>&alpha;</sub> and V<sub>&beta;</sub> voltages and outputs corresponding space vector modulation voltages.</p>
      mask Display: fprintf('Space\n Vector\n Generation');
  Subsystem2 : Subsystem  mask(Clarke Transform){}
      mask help:
      | <p>Compute Clarke transformation on balanced 3-phase inputs into balanced 2-phase orthogonal outputs.
      | <br>
      | <br>
      | The block accepts two signals out of three phases, and outputs corresponding &alpha;-&beta; axis components, where phase-a axis is aligned with alpha axis.</p>
      mask Display: fprintf('Clarke\nTransform');
  Subsystem3 : Subsystem  mask(Park Transform){AxisAlignment=D-axis}
      mask prompts: AxisAlignment "Alpha (phase-a) axis alignment:"
      mask help:
      | <p>Compute Park transformation on stationary reference frame inputs into rotating reference frame outputs.
      | <br><br>
      | The block accepts the following:
      | <ul>
      |   <li>&alpha;-&beta; axis components in stationary reference frame</li>
      |   <li>Sine and cosine values of corresponding angle of transformation</li>
      | </ul>
      | The block outputs direct and quadrature axis components in rotating reference frame.
      | <br><br>
      | D-axis alignment with alpha (phase-a) is popular in motor control theory while Q-axis alignment with alpha (phase-a) is more suitable for power conversion applications.</p>
      mask init:
      | dlgSett.Offset = 0;
      | 
      | switch AxisAlignment
      |     case 'Q-axis'
      |         dlgSett.Offset = 90;
      |     case 'D-axis'
      |         dlgSett.Offset = 0;
      |     otherwise
      | end
      mask TypeOptions AxisAlignment: D-axis | Q-axis
      mask Display: fprintf('Park\nTransform');
  Subsystem4 : Subsystem  mask(Inverse Park Transform){AxisAlignment=D-axis}
      mask prompts: AxisAlignment "Alpha (phase-a ) axis alignment:"
      mask help:
      | <p>Compute Inverse Park transformation on rotating reference frame inputs into stationary reference frame outputs.
      | <br><br>
      | The block accepts the following:
      | <ul>
      | <li>d-q axis components in rotating reference frame</li>
      | <li>Sine and cosine values of corresponding angle of transformation</li>
      | </ul>
      | The block outputs &alpha;-&beta; axis components in stationary reference frame.
      | <br><br>
      | D-axis alignment with alpha (phase-a) is popular in motor control theory while Q-axis alignment with alpha (phase-a) is more suitable for power conversion applications.</p>
      mask init:
      | dlgSett.Offset = 0;
      | 
      | switch AxisAlignment
      |     case 'Q-axis'
      |         dlgSett.Offset = 90;
      |     case 'D-axis'
      |         dlgSett.Offset = 0;
      |     otherwise
      | end
      mask TypeOptions AxisAlignment: D-axis | Q-axis
      mask Display: fprintf('Inverse Park\n Transform');
  deadzone_comp : MATLAB Function  TreatAsAtomicUnit=on
  Out1 : Outport
  wires:
  Subsystem3/2(Qs) -> Current_Controllers1/5(q_current_measured (A))
  deadzone_comp/1(Ta) -> Mux1/1
  Sine-Cosine Lookup/1(sin) -> [sinTheta], Subsystem3/3(sine)
  deadzone_comp/2(Tb) -> Mux1/2
  Demux/2 -> Subsystem2/2(b)
  Subsystem4/2(Beta) -> Subsystem1/2(Beta)
  [cosTheta] -> Subsystem4/4(cos)
  Subsystem/1(d_current_command) -> Current_Controllers1/2(d_current_command (A))
  Subsystem1/2(Tb) -> deadzone_comp/2(TbI)
  Sine-Cosine Lookup/2(cos) -> [cosTheta], Subsystem3/4(cos)
  Bus Selector1/2 -> Subsystem4/2(Qs)  "<quadrature_voltage>"
  Enum_To_Int/1 -> Detect_Change/1
  Subsystem4/1(Alpha) -> Subsystem1/1(Alpha)
  Subsystem1/3(Tc) -> deadzone_comp/3(TcI)
  controller_mode/1 -> Enum_To_Int/1
  q_current_command (A)1/1 -> Current_Controllers1/3(q_current_command (A))
  Iab_fb/1 -> Demux/1
  Data Store Read1/1 -> Logical Operator/1
  Mux1/1 -> Out1/1
  Current_Controllers1/1(dq_axis_voltages (V)) -> Bus Selector1/1
  Speed/1 -> Current_Controllers1/6(Electrical_speed_measured)
  Subsystem3/1(Ds) -> Current_Controllers1/4(d_current_measured (A))
  Subsystem1/1(Ta) -> deadzone_comp/1(TaI)
  Detect_Change/1 -> OR/2
  Bus Selector1/1 -> Subsystem4/1(Ds)  "<direct_voltage>"
  Logical Operator/1 -> OR/1
  deadzone_comp/3(Tc) -> Mux1/3
  OR/1 -> Current_Controllers1/1(reset_integrators)
  [sinTheta] -> Subsystem4/3(sin)
  Demux/1 -> Subsystem2/1(a)
  Subsystem2/2(Beta) -> Subsystem3/2(Beta)
  Subsystem2/1(Alpha) -> Subsystem3/1(Alpha)
  Feedback/1 -> Sine-Cosine Lookup/1(Theta)
